simulink model "P6_filter"  (R2020b)
settings: Solver=VariableStepAuto  StartTime=0.0  StopTime=10.0  RelTol=1e-3
libraries: simulink x1
settings Model: Creator=mluser  LastModifiedBy=mluser

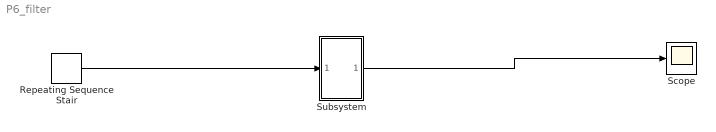
== system P6_filter ==
  Repeating Sequence Stair : simulink/Sources/Repeating Sequence Stair  OutValues=[3 1 4 2 1].'  tsamp=-1  OutMin=[]  OutMax=[]  OutDataTypeStr=double  OutputDataTypeScalingMode=double  OutDataType=fixdt(0,8)  ConRadixGroup=Best Precision: Vector-wise  OutScaling=2^-12
  Scope : Scope
  Subsystem : Subsystem
  wires:
  Repeating Sequence Stair/1 -> Subsystem/1(In1)
  Subsystem/1(Out1) -> Scope/1

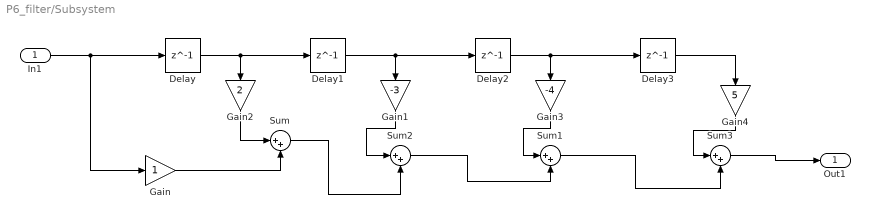
== system P6_filter/Subsystem ==
  In1 : Inport
  Delay{,1..3} (4 alike) : Delay  DelayLength=1
  Gain : Gain
  Gain1 : Gain  Gain=-3
  Gain2 : Gain  Gain=2
  Gain3 : Gain  Gain=-4
  Gain4 : Gain  Gain=5
  Sum{,1..3} (4 alike) : Sum  Inputs=|++
  Out1 : Outport
  wires:
  Gain/1 -> Sum/2
  Gain4/1 -> Sum3/1
  Sum/1 -> Sum2/2
  Sum3/1 -> Out1/1
  Sum1/1 -> Sum3/2
  Gain2/1 -> Sum/1
  Delay1/1 -> Delay2/1, Gain1/1
  Gain3/1 -> Sum1/1
  Delay2/1 -> Delay3/1, Gain3/1
  Delay/1 -> Delay1/1, Gain2/1
  In1/1 -> Gain/1, Delay/1
  Sum2/1 -> Sum1/2
  Delay3/1 -> Gain4/1
  Gain1/1 -> Sum2/1
